simulink model "nn_fuel_control_3_10"  (R2021a)
settings: Solver=ode15s  StartTime=0.0  StopTime=T  MaxStep=.01  RelTol=1e-3
undefined symbols (not defined in the file): AF_sensor_tol, fault_time, fuel_inj_tol, kappa_tol, MAF_sensor_tol, pump_tol, tau_ww_tol
libraries: neural x70
(part 3 of 3)

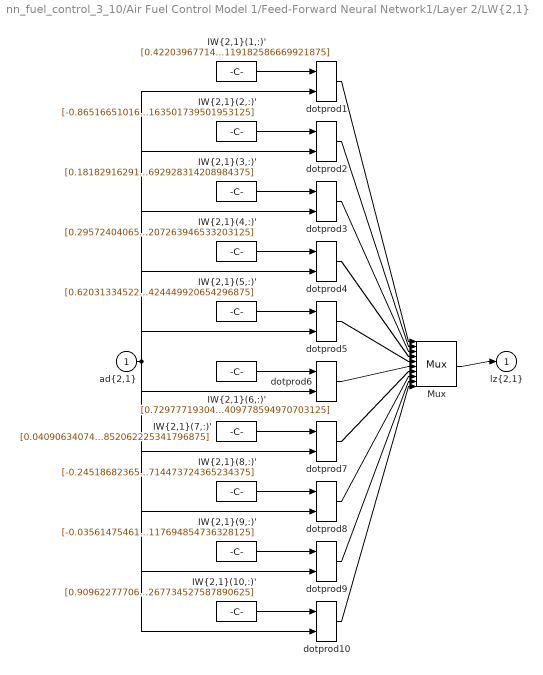
== system nn_fuel_control_3_10/Air Fuel Control Model 1/Feed-Forward Neural Network1/Layer 2/LW{2,1} ==
  "ad{2,1}" : Inport  PortDimensions=10
      mask Display: e = 0.06;c1 = [120 230 180]/255;c2 = ([120 230 180]+0)/(256+128);c3 = ([120 230 180]+128)/(256+128);patch([0 1 1 0],[0 0 1 1],c1);patch([0 1 1 1-e 1-e 0+e],[0 0 1 1-e 0+e 0+e],c2);patch([0 0 1 1-e 0+e 0+e],[0 1 1 1-e 1-e 0+e],c3);plot([0 1 1 0 0],[0 0 1 1 0]);
  "IW{2,1}(1,:)'" : Constant  Value=[0.422039677146083092029726913096965290606021881103515625;-0.110092252616240227069965840200893580913543701171875;-0.26250402610766976341238887471263296902179718017578125;-0.0048946197898318555274954633205197751522064208984375;-0.32867619613755272300892329440102912485599517822265625;0.902942789239071341711451168521307408809661865234375;0.4878626703089585792127991226152516901493072509765625;0.617102583012261174388868312234990298748016357421875;0.733631816964918304080356392660178244113922119140625;0.394170838499643849672793294303119182586669921875]
      mask Display: e = 0.06;c1 = [120 150 230]/255;c2 = ([120 150 230]+0)/383;c3 = ([120 150 230]+128)/383;patch([0 1 1 0],[0 0 1 1],c1);patch([0 1 1 1-e 1-e 0+e],[0 0 1 1-e 0+e 0+e],c2);patch([0 0 1 1-e 0+e 0+e],[0 1 1 1-e 1-e 0+e],c3);plot([0 1 1 0 0],[0 0 1 1 0]);disp('weights');
  "IW{2,1}(10,:)'" : Constant  Value=[0.90962277706535576982105339993722736835479736328125;-0.6963449514150970021120201636222191154956817626953125;0.01080664673637077299872544244863092899322509765625;0.3356832194814760583767565549351274967193603515625;-0.8333879786409565948446243055514059960842132568359375;0.0388654008517956839341422892175614833831787109375;-0.876991458324715811301075518713332712650299072265625;0.2552200485621887171561184004531241953372955322265625;0.439737074727967414133900092565454542636871337890625;-0.454907616285860516569528044783510267734527587890625]
      mask Display: e = 0.06;c1 = [120 150 230]/255;c2 = ([120 150 230]+0)/383;c3 = ([120 150 230]+128)/383;patch([0 1 1 0],[0 0 1 1],c1);patch([0 1 1 1-e 1-e 0+e],[0 0 1 1-e 0+e 0+e],c2);patch([0 0 1 1-e 0+e 0+e],[0 1 1 1-e 1-e 0+e],c3);plot([0 1 1 0 0],[0 0 1 1 0]);disp('weights');
  "IW{2,1}(2,:)'" : Constant  Value=[-0.8651665101614505193339255129103548824787139892578125;-0.68113174408582732866079822997562587261199951171875;0.8404892436305388958572848423500545322895050048828125;0.6586664029004605236394809253397397696971893310546875;-0.7731369627331130534031444767606444656848907470703125;-0.8362478809265689871921267695142887532711029052734375;0.81195057507577839128742880347999744117259979248046875;0.64588522595887110089307725502294488251209259033203125;-0.1523813423040767389693428413011133670806884765625;0.9829939123414395130140519540873356163501739501953125]
      mask Display: e = 0.06;c1 = [120 150 230]/255;c2 = ([120 150 230]+0)/383;c3 = ([120 150 230]+128)/383;patch([0 1 1 0],[0 0 1 1],c1);patch([0 1 1 1-e 1-e 0+e],[0 0 1 1-e 0+e 0+e],c2);patch([0 0 1 1-e 0+e 0+e],[0 1 1 1-e 1-e 0+e],c3);plot([0 1 1 0 0],[0 0 1 1 0]);disp('weights');
  "IW{2,1}(3,:)'" : Constant  Value=[0.181829162913355713016017034533433616161346435546875;-0.881434984567488921669564660987816751003265380859375;-0.1876417286710629905854830212774686515331268310546875;-0.8571525749339719002506399192498065531253814697265625;-0.482981460609078538936955737881362438201904296875;0.56940545520623420117090063286013901233673095703125;0.0259222786987063358310479088686406612396240234375;0.4738233938363729524922973723732866346836090087890625;-0.040986332132006086936826250166632235050201416015625;-0.8081043995213919028941518263309262692928314208984375]
      mask Display: e = 0.06;c1 = [120 150 230]/255;c2 = ([120 150 230]+0)/383;c3 = ([120 150 230]+128)/383;patch([0 1 1 0],[0 0 1 1],c1);patch([0 1 1 1-e 1-e 0+e],[0 0 1 1-e 0+e 0+e],c2);patch([0 0 1 1-e 0+e 0+e],[0 1 1 1-e 1-e 0+e],c3);plot([0 1 1 0 0],[0 0 1 1 0]);disp('weights');
  "IW{2,1}(4,:)'" : Constant  Value=[0.295724040659893938620683684348477981984615325927734375;-0.3268515229616741901708110162871889770030975341796875;-0.279057639543601521125992803717963397502899169921875;0.79686882507062062330760454642586410045623779296875;0.0661197066964048507653473052414483390748500823974609375;-0.63298798947408829729255330676096491515636444091796875;0.1316826637177681558199537903419695794582366943359375;-0.1431159471639171509860233300059917382895946502685546875;0.9243644520376523843196991947479546070098876953125;-0.71110368735452045285683198017068207263946533203125]
      mask Display: e = 0.06;c1 = [120 150 230]/255;c2 = ([120 150 230]+0)/383;c3 = ([120 150 230]+128)/383;patch([0 1 1 0],[0 0 1 1],c1);patch([0 1 1 1-e 1-e 0+e],[0 0 1 1-e 0+e 0+e],c2);patch([0 0 1 1-e 0+e 0+e],[0 1 1 1-e 1-e 0+e],c3);plot([0 1 1 0 0],[0 0 1 1 0]);disp('weights');
  "IW{2,1}(5,:)'" : Constant  Value=[0.6203133452260793934129878834937699139118194580078125;0.901635231669291048461900572874583303928375244140625;-0.3287366297786744606668207779875956475734710693359375;-0.1271174786615658636179659879417158663272857666015625;-0.8464951772599962342980006724246777594089508056640625;0.28518177033808012055260405759327113628387451171875;0.513679542182248649595521783339790999889373779296875;0.6428584550354512483494318075827322900295257568359375;-0.4251606596384103209373961362871341407299041748046875;-0.27453898190018133362855223822407424449920654296875]
      mask Display: e = 0.06;c1 = [120 150 230]/255;c2 = ([120 150 230]+0)/383;c3 = ([120 150 230]+128)/383;patch([0 1 1 0],[0 0 1 1],c1);patch([0 1 1 1-e 1-e 0+e],[0 0 1 1-e 0+e 0+e],c2);patch([0 0 1 1-e 0+e 0+e],[0 1 1 1-e 1-e 0+e],c3);plot([0 1 1 0 0],[0 0 1 1 0]);disp('weights');
  "IW{2,1}(6,:)'" : Constant  Value=[0.7297771930479635127397841642959974706172943115234375;0.23165854469143543070686064311303198337554931640625;0.96494142671238758435237059529754333198070526123046875;-0.390555914482942245768981592846103012561798095703125;-0.90514919206743993385089197545312345027923583984375;-0.438431277886345449612548463846906088292598724365234375;-0.0802142409019130919745066421455703675746917724609375;0.575344599813421897493981305160559713840484619140625;0.1934076537033260212439245151472277939319610595703125;0.934934713944724382628237435710616409778594970703125]
      mask Display: e = 0.06;c1 = [120 150 230]/255;c2 = ([120 150 230]+0)/383;c3 = ([120 150 230]+128)/383;patch([0 1 1 0],[0 0 1 1],c1);patch([0 1 1 1-e 1-e 0+e],[0 0 1 1-e 0+e 0+e],c2);patch([0 0 1 1-e 0+e 0+e],[0 1 1 1-e 1-e 0+e],c3);plot([0 1 1 0 0],[0 0 1 1 0]);disp('weights');
  "IW{2,1}(7,:)'" : Constant  Value=[0.040906340743202616871965204836669727228581905364990234375;0.3152445102858461023487279817345552146434783935546875;-0.96641677936879866184227694247965700924396514892578125;0.858094101605435977120350798941217362880706787109375;0.50777822108413539492488553150906227529048919677734375;-0.19512639085175231823399144559516571462154388427734375;-0.66692474021244618764825418111286126077175140380859375;0.280350917189209847268926978358649648725986480712890625;-0.696901686135316111858628573827445507049560546875;0.326149132414730313911377379554323852062225341796875]
      mask Display: e = 0.06;c1 = [120 150 230]/255;c2 = ([120 150 230]+0)/383;c3 = ([120 150 230]+128)/383;patch([0 1 1 0],[0 0 1 1],c1);patch([0 1 1 1-e 1-e 0+e],[0 0 1 1-e 0+e 0+e],c2);patch([0 0 1 1-e 0+e 0+e],[0 1 1 1-e 1-e 0+e],c3);plot([0 1 1 0 0],[0 0 1 1 0]);disp('weights');
  "IW{2,1}(8,:)'" : Constant  Value=[-0.245186823656732055809470693930052220821380615234375;0.2891152018195357609187112757354043424129486083984375;0.743202086592667843234494284843094646930694580078125;0.3425737123726282362667916459031403064727783203125;-0.057163964796326904860279682907275855541229248046875;-0.3148850353591388095964020976680330932140350341796875;-0.160467488716616646371448950958438217639923095703125;-0.9476340821065243336107641880516894161701202392578125;0.223274479885884336027856988948769867420196533203125;-0.993767070952779274506383444531820714473724365234375]
      mask Display: e = 0.06;c1 = [120 150 230]/255;c2 = ([120 150 230]+0)/383;c3 = ([120 150 230]+128)/383;patch([0 1 1 0],[0 0 1 1],c1);patch([0 1 1 1-e 1-e 0+e],[0 0 1 1-e 0+e 0+e],c2);patch([0 0 1 1-e 0+e 0+e],[0 1 1 1-e 1-e 0+e],c3);plot([0 1 1 0 0],[0 0 1 1 0]);disp('weights');
  "IW{2,1}(9,:)'" : Constant  Value=[-0.035614754618427287014004178899995167739689350128173828125;0.1634174485713522084751048168982379138469696044921875;-0.03107010615764423111517800180081394501030445098876953125;-0.0735264940139603861979367138701491057872772216796875;0.455642930383942879046799134812317788600921630859375;-0.70351463548461057317950917422422207891941070556640625;0.04472929077745153858547411118706804700195789337158203125;-0.77337147245237236603543351520784199237823486328125;-0.103734070298024949607906819437630474567413330078125;-0.556461539732368226651715303887613117694854736328125]
      mask Display: e = 0.06;c1 = [120 150 230]/255;c2 = ([120 150 230]+0)/383;c3 = ([120 150 230]+128)/383;patch([0 1 1 0],[0 0 1 1],c1);patch([0 1 1 1-e 1-e 0+e],[0 0 1 1-e 0+e 0+e],c2);patch([0 0 1 1-e 0+e 0+e],[0 1 1 1-e 1-e 0+e],c3);plot([0 1 1 0 0],[0 0 1 1 0]);disp('weights');
  Mux : Mux  Inputs=10
      mask Display: e = 0.06;c1 = [120 150 230]/255;c2 = ([120 150 230]+0)/383;c3 = ([120 150 230]+128)/383;patch([0 1 1 0],[0 0 1 1],c1);patch([0 1 1 1-e 1-e 0+e],[0 0 1 1-e 0+e 0+e],c2);patch([0 0 1 1-e 0+e 0+e],[0 1 1 1-e 1-e 0+e],c3);plot([0 1 1 0 0],[0 0 1 1 0]);disp('Mux');
  dotprod{1..10} (10 alike) : neural/Weight Functions/dotprod
  "lz{2,1}" : Outport
      mask Display: e = 0.06;c1 = [120 230 180]/255;c2 = ([120 230 180]+0)/(256+128);c3 = ([120 230 180]+128)/(256+128);patch([0 1 1 0],[0 0 1 1],c1);patch([0 1 1 1-e 1-e 0+e],[0 0 1 1-e 0+e 0+e],c2);patch([0 0 1 1-e 0+e 0+e],[0 1 1 1-e 1-e 0+e],c3);plot([0 1 1 0 0],[0 0 1 1 0]);
  wires:
  "IW{2,1}(1,:)'"/1 -> dotprod1/1
  "ad{2,1}"/1 -> dotprod1/2, dotprod2/2, dotprod3/2, dotprod4/2, dotprod5/2, dotprod6/2, dotprod7/2, dotprod8/2, dotprod9/2, dotprod10/2
  dotprod1/1 -> Mux/1
  "IW{2,1}(2,:)'"/1 -> dotprod2/1
  dotprod2/1 -> Mux/2
  "IW{2,1}(3,:)'"/1 -> dotprod3/1
  dotprod3/1 -> Mux/3
  "IW{2,1}(4,:)'"/1 -> dotprod4/1
  dotprod4/1 -> Mux/4
  "IW{2,1}(5,:)'"/1 -> dotprod5/1
  dotprod5/1 -> Mux/5
  "IW{2,1}(6,:)'"/1 -> dotprod6/1
  dotprod6/1 -> Mux/6
  "IW{2,1}(7,:)'"/1 -> dotprod7/1
  dotprod7/1 -> Mux/7
  "IW{2,1}(8,:)'"/1 -> dotprod8/1
  dotprod8/1 -> Mux/8
  "IW{2,1}(9,:)'"/1 -> dotprod9/1
  dotprod9/1 -> Mux/9
  "IW{2,1}(10,:)'"/1 -> dotprod10/1
  dotprod10/1 -> Mux/10
  Mux/1 -> "lz{2,1}"/1

== system nn_fuel_control_3_10/Air Fuel Control Model 1/Feed-Forward Neural Network1/Layer 3/Delays 1 ==
  "p{3}" : Inport  PortDimensions=10
      mask Display: e = 0.06;c1 = [120 230 180]/255;c2 = ([120 230 180]+0)/(256+128);c3 = ([120 230 180]+128)/(256+128);patch([0 1 1 0],[0 0 1 1],c1);patch([0 1 1 1-e 1-e 0+e],[0 0 1 1-e 0+e 0+e],c2);patch([0 0 1 1-e 0+e 0+e],[0 1 1 1-e 1-e 0+e],c3);plot([0 1 1 0 0],[0 0 1 1 0]);
  mux : Mux  Inputs=1
      mask Display: e = 0.06;c1 = [120 150 230]/255;c2 = ([120 150 230]+0)/383;c3 = ([120 150 230]+128)/383;patch([0 1 1 0],[0 0 1 1],c1);patch([0 1 1 1-e 1-e 0+e],[0 0 1 1-e 0+e 0+e],c2);patch([0 0 1 1-e 0+e 0+e],[0 1 1 1-e 1-e 0+e],c3);plot([0 1 1 0 0],[0 0 1 1 0]);disp('Mux')
  "pd{3,2}" : Outport
      mask Display: e = 0.06;c1 = [120 230 180]/255;c2 = ([120 230 180]+0)/(256+128);c3 = ([120 230 180]+128)/(256+128);patch([0 1 1 0],[0 0 1 1],c1);patch([0 1 1 1-e 1-e 0+e],[0 0 1 1-e 0+e 0+e],c2);patch([0 0 1 1-e 0+e 0+e],[0 1 1 1-e 1-e 0+e],c3);plot([0 1 1 0 0],[0 0 1 1 0]);
  wires:
  "p{3}"/1 -> mux/1
  mux/1 -> "pd{3,2}"/1

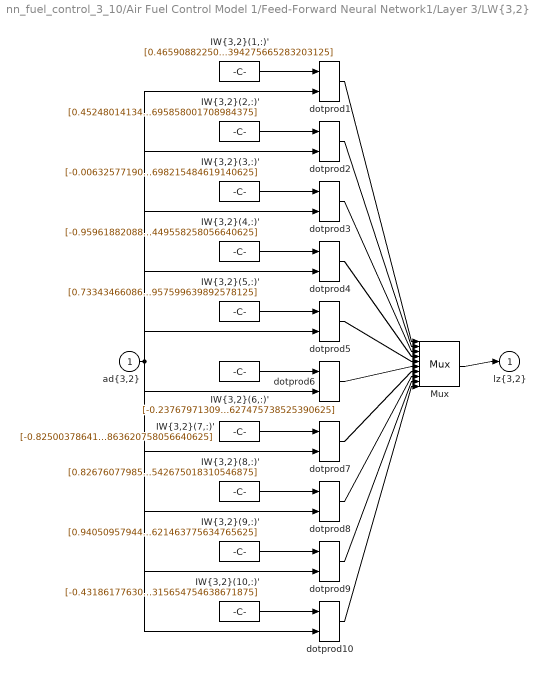
== system nn_fuel_control_3_10/Air Fuel Control Model 1/Feed-Forward Neural Network1/Layer 3/LW{3,2} ==
  "ad{3,2}" : Inport  PortDimensions=10
      mask Display: e = 0.06;c1 = [120 230 180]/255;c2 = ([120 230 180]+0)/(256+128);c3 = ([120 230 180]+128)/(256+128);patch([0 1 1 0],[0 0 1 1],c1);patch([0 1 1 1-e 1-e 0+e],[0 0 1 1-e 0+e 0+e],c2);patch([0 0 1 1-e 0+e 0+e],[0 1 1 1-e 1-e 0+e],c3);plot([0 1 1 0 0],[0 0 1 1 0]);
  "IW{3,2}(1,:)'" : Constant  Value=[0.465908822500017583134734877603477798402309417724609375;-0.413487608206142664979410028536221943795680999755859375;-0.25595023125727589530242767068557441234588623046875;0.79533255427383819924358476782799698412418365478515625;-0.3198554688185104577513584445114247500896453857421875;-0.26425170262540387255967289092950522899627685546875;-0.96446227621692859344193493598140776157379150390625;0.1110265066473614670172764817834831774234771728515625;0.22084634591132246139721928557264618575572967529296875;-0.0783795812571821404191041438025422394275665283203125]
      mask Display: e = 0.06;c1 = [120 150 230]/255;c2 = ([120 150 230]+0)/383;c3 = ([120 150 230]+128)/383;patch([0 1 1 0],[0 0 1 1],c1);patch([0 1 1 1-e 1-e 0+e],[0 0 1 1-e 0+e 0+e],c2);patch([0 0 1 1-e 0+e 0+e],[0 1 1 1-e 1-e 0+e],c3);plot([0 1 1 0 0],[0 0 1 1 0]);disp('weights');
  "IW{3,2}(10,:)'" : Constant  Value=[-0.4318617763054584113291411995305679738521575927734375;-0.032997678117612373738243292109473259188234806060791015625;0.077801025420537239796203721198253333568572998046875;-0.28911309780956695458797867104294709861278533935546875;-0.276713333572291997342063041287474334239959716796875;-0.263564907235820322650710068046464584767818450927734375;-0.51348229867116312874486538930796086788177490234375;-0.6075701084650637628925551325664855539798736572265625;-0.1908663702211096657723743419410311616957187652587890625;0.502134394339247336347398231737315654754638671875]
      mask Display: e = 0.06;c1 = [120 150 230]/255;c2 = ([120 150 230]+0)/383;c3 = ([120 150 230]+128)/383;patch([0 1 1 0],[0 0 1 1],c1);patch([0 1 1 1-e 1-e 0+e],[0 0 1 1-e 0+e 0+e],c2);patch([0 0 1 1-e 0+e 0+e],[0 1 1 1-e 1-e 0+e],c3);plot([0 1 1 0 0],[0 0 1 1 0]);disp('weights');
  "IW{3,2}(2,:)'" : Constant  Value=[0.452480141341178032643455253491993062198162078857421875;0.336080692249946688665573901744210161268711090087890625;-0.750580224709083143608268073876388370990753173828125;-0.52823687812015529541298519689007662236690521240234375;0.602301465570855842912578737013973295688629150390625;0.63024563212891104857504842584603466093540191650390625;-0.356127133216790958680775247557903639972209930419921875;-0.036352884411245955931235585012473165988922119140625;0.291588369681691716994720309230615384876728057861328125;0.1676526656541683646395313189714215695858001708984375]
      mask Display: e = 0.06;c1 = [120 150 230]/255;c2 = ([120 150 230]+0)/383;c3 = ([120 150 230]+128)/383;patch([0 1 1 0],[0 0 1 1],c1);patch([0 1 1 1-e 1-e 0+e],[0 0 1 1-e 0+e 0+e],c2);patch([0 0 1 1-e 0+e 0+e],[0 1 1 1-e 1-e 0+e],c3);plot([0 1 1 0 0],[0 0 1 1 0]);disp('weights');
  "IW{3,2}(3,:)'" : Constant  Value=[-0.0063257719015989977151548373512923717498779296875;0.1558232650998754298399262552266009151935577392578125;0.21356467202521312032104106037877500057220458984375;-0.5606276936605281147052437518141232430934906005859375;0.51247289446128529988300215336494147777557373046875;-0.6789132841767884229966512066312134265899658203125;-0.105704557253306408171056318678893148899078369140625;-0.0089827216141546983863008790649473667144775390625;0.010488749062883329088435857556760311126708984375;0.1097273920785470924244009438552893698215484619140625]
      mask Display: e = 0.06;c1 = [120 150 230]/255;c2 = ([120 150 230]+0)/383;c3 = ([120 150 230]+128)/383;patch([0 1 1 0],[0 0 1 1],c1);patch([0 1 1 1-e 1-e 0+e],[0 0 1 1-e 0+e 0+e],c2);patch([0 0 1 1-e 0+e 0+e],[0 1 1 1-e 1-e 0+e],c3);plot([0 1 1 0 0],[0 0 1 1 0]);disp('weights');
  "IW{3,2}(4,:)'" : Constant  Value=[-0.9596188208888793980122500215657055377960205078125;-0.8746551071446122538333156626322306692600250244140625;-0.1240862576936716532571836069109849631786346435546875;-0.9366084767927647103391564087360166013240814208984375;-0.2263567918631845810040204014512710273265838623046875;-0.7551613682655489157014017109759151935577392578125;-0.0137802781081342029523284509195946156978607177734375;0.978542105587190125248753247433342039585113525390625;-0.1979323813352078520466648114961571991443634033203125;0.636282512328963267833614736446179449558258056640625]
      mask Display: e = 0.06;c1 = [120 150 230]/255;c2 = ([120 150 230]+0)/383;c3 = ([120 150 230]+128)/383;patch([0 1 1 0],[0 0 1 1],c1);patch([0 1 1 1-e 1-e 0+e],[0 0 1 1-e 0+e 0+e],c2);patch([0 0 1 1-e 0+e 0+e],[0 1 1 1-e 1-e 0+e],c3);plot([0 1 1 0 0],[0 0 1 1 0]);disp('weights');
  "IW{3,2}(5,:)'" : Constant  Value=[0.73343466086165565176457903362461365759372711181640625;0.960980758123656908509246932226233184337615966796875;-0.134217532509697701215145571040920913219451904296875;0.11442774545926277796059622460234095342457294464111328125;0.6723741038002055692146541332476772367954254150390625;0.1438551765328461851112251679296605288982391357421875;0.9363889336038428989894555343198589980602264404296875;0.137441760075660557305354814161546528339385986328125;-0.8843285718670441664102099821320734918117523193359375;0.5522017606648639276301082645659334957599639892578125]
      mask Display: e = 0.06;c1 = [120 150 230]/255;c2 = ([120 150 230]+0)/383;c3 = ([120 150 230]+128)/383;patch([0 1 1 0],[0 0 1 1],c1);patch([0 1 1 1-e 1-e 0+e],[0 0 1 1-e 0+e 0+e],c2);patch([0 0 1 1-e 0+e 0+e],[0 1 1 1-e 1-e 0+e],c3);plot([0 1 1 0 0],[0 0 1 1 0]);disp('weights');
  "IW{3,2}(6,:)'" : Constant  Value=[-0.2376797130922718437329166363269905559718608856201171875;-0.3245060471454490613751886485260911285877227783203125;0.411253730585999566216059974976815283298492431640625;0.3281032645082484489051921627833507955074310302734375;-0.5180651518724077586597331901430152356624603271484375;-0.5577078697023740705418504148838110268115997314453125;-0.422261332231368469170007529100985266268253326416015625;-0.070689711751910966341938546975143253803253173828125;-0.1758320370175628089004504772674408741295337677001953125;0.7513529749619716202602148769074119627475738525390625]
      mask Display: e = 0.06;c1 = [120 150 230]/255;c2 = ([120 150 230]+0)/383;c3 = ([120 150 230]+128)/383;patch([0 1 1 0],[0 0 1 1],c1);patch([0 1 1 1-e 1-e 0+e],[0 0 1 1-e 0+e 0+e],c2);patch([0 0 1 1-e 0+e 0+e],[0 1 1 1-e 1-e 0+e],c3);plot([0 1 1 0 0],[0 0 1 1 0]);disp('weights');
  "IW{3,2}(7,:)'" : Constant  Value=[-0.82500378641395910594980023233802057802677154541015625;0.96291679796392204426780381254502572119235992431640625;0.5803596168647000563822757612797431647777557373046875;-0.2701456506325394801848460701876319944858551025390625;0.8890348593138062138763189068413339555263519287109375;0.1501557516428747851566782856025383807718753814697265625;0.481666771587706765700431787990964949131011962890625;-0.7831361801558021085156724439002573490142822265625;-0.026613027462942674683521460110569023527204990386962890625;-0.1646446034291531024251753478893078863620758056640625]
      mask Display: e = 0.06;c1 = [120 150 230]/255;c2 = ([120 150 230]+0)/383;c3 = ([120 150 230]+128)/383;patch([0 1 1 0],[0 0 1 1],c1);patch([0 1 1 1-e 1-e 0+e],[0 0 1 1-e 0+e 0+e],c2);patch([0 0 1 1-e 0+e 0+e],[0 1 1 1-e 1-e 0+e],c3);plot([0 1 1 0 0],[0 0 1 1 0]);disp('weights');
  "IW{3,2}(8,:)'" : Constant  Value=[0.82676077985266804848407673489418812096118927001953125;-0.87879337999093143363182889515883289277553558349609375;-0.8573989414424232347045062851975671947002410888671875;0.6488948308169446566040505786077119410037994384765625;0.841872789003470956004093750379979610443115234375;-0.55549591509967577440676222977344878017902374267578125;0.59327158091704268461086257957504130899906158447265625;0.369291055697225534260041968082077801227569580078125;0.89098865986625153112754560424946248531341552734375;0.945757196895765428479307956877164542675018310546875]
      mask Display: e = 0.06;c1 = [120 150 230]/255;c2 = ([120 150 230]+0)/383;c3 = ([120 150 230]+128)/383;patch([0 1 1 0],[0 0 1 1],c1);patch([0 1 1 1-e 1-e 0+e],[0 0 1 1-e 0+e 0+e],c2);patch([0 0 1 1-e 0+e 0+e],[0 1 1 1-e 1-e 0+e],c3);plot([0 1 1 0 0],[0 0 1 1 0]);disp('weights');
  "IW{3,2}(9,:)'" : Constant  Value=[0.9405095794473343762120975952711887657642364501953125;-0.188806428409112159183536050477414391934871673583984375;0.8350720698739089176143579607014544308185577392578125;0.2144367638571101630784454528111382387578487396240234375;-0.3297992370033802078665985391126014292240142822265625;0.00879039483057554062173100106747369864024221897125244140625;0.66039899729722628674011275506927631795406341552734375;-0.3996949053173801669203157871379517018795013427734375;-0.90049767130397506686989572699530981481075286865234375;-0.0075342401012241655422485564486123621463775634765625]
      mask Display: e = 0.06;c1 = [120 150 230]/255;c2 = ([120 150 230]+0)/383;c3 = ([120 150 230]+128)/383;patch([0 1 1 0],[0 0 1 1],c1);patch([0 1 1 1-e 1-e 0+e],[0 0 1 1-e 0+e 0+e],c2);patch([0 0 1 1-e 0+e 0+e],[0 1 1 1-e 1-e 0+e],c3);plot([0 1 1 0 0],[0 0 1 1 0]);disp('weights');
  Mux : Mux  Inputs=10
      mask Display: e = 0.06;c1 = [120 150 230]/255;c2 = ([120 150 230]+0)/383;c3 = ([120 150 230]+128)/383;patch([0 1 1 0],[0 0 1 1],c1);patch([0 1 1 1-e 1-e 0+e],[0 0 1 1-e 0+e 0+e],c2);patch([0 0 1 1-e 0+e 0+e],[0 1 1 1-e 1-e 0+e],c3);plot([0 1 1 0 0],[0 0 1 1 0]);disp('Mux');
  dotprod{1..10} (10 alike) : neural/Weight Functions/dotprod
  "lz{3,2}" : Outport
      mask Display: e = 0.06;c1 = [120 230 180]/255;c2 = ([120 230 180]+0)/(256+128);c3 = ([120 230 180]+128)/(256+128);patch([0 1 1 0],[0 0 1 1],c1);patch([0 1 1 1-e 1-e 0+e],[0 0 1 1-e 0+e 0+e],c2);patch([0 0 1 1-e 0+e 0+e],[0 1 1 1-e 1-e 0+e],c3);plot([0 1 1 0 0],[0 0 1 1 0]);
  wires:
  "IW{3,2}(1,:)'"/1 -> dotprod1/1
  "ad{3,2}"/1 -> dotprod1/2, dotprod2/2, dotprod3/2, dotprod4/2, dotprod5/2, dotprod6/2, dotprod7/2, dotprod8/2, dotprod9/2, dotprod10/2
  dotprod1/1 -> Mux/1
  "IW{3,2}(2,:)'"/1 -> dotprod2/1
  dotprod2/1 -> Mux/2
  "IW{3,2}(3,:)'"/1 -> dotprod3/1
  dotprod3/1 -> Mux/3
  "IW{3,2}(4,:)'"/1 -> dotprod4/1
  dotprod4/1 -> Mux/4
  "IW{3,2}(5,:)'"/1 -> dotprod5/1
  dotprod5/1 -> Mux/5
  "IW{3,2}(6,:)'"/1 -> dotprod6/1
  dotprod6/1 -> Mux/6
  "IW{3,2}(7,:)'"/1 -> dotprod7/1
  dotprod7/1 -> Mux/7
  "IW{3,2}(8,:)'"/1 -> dotprod8/1
  dotprod8/1 -> Mux/8
  "IW{3,2}(9,:)'"/1 -> dotprod9/1
  dotprod9/1 -> Mux/9
  "IW{3,2}(10,:)'"/1 -> dotprod10/1
  dotprod10/1 -> Mux/10
  Mux/1 -> "lz{3,2}"/1

== system nn_fuel_control_3_10/Air Fuel Control Model 1/Feed-Forward Neural Network1/Layer 4/Delays 1 ==
  "p{4}" : Inport  PortDimensions=10
      mask Display: e = 0.06;c1 = [120 230 180]/255;c2 = ([120 230 180]+0)/(256+128);c3 = ([120 230 180]+128)/(256+128);patch([0 1 1 0],[0 0 1 1],c1);patch([0 1 1 1-e 1-e 0+e],[0 0 1 1-e 0+e 0+e],c2);patch([0 0 1 1-e 0+e 0+e],[0 1 1 1-e 1-e 0+e],c3);plot([0 1 1 0 0],[0 0 1 1 0]);
  mux : Mux  Inputs=1
      mask Display: e = 0.06;c1 = [120 150 230]/255;c2 = ([120 150 230]+0)/383;c3 = ([120 150 230]+128)/383;patch([0 1 1 0],[0 0 1 1],c1);patch([0 1 1 1-e 1-e 0+e],[0 0 1 1-e 0+e 0+e],c2);patch([0 0 1 1-e 0+e 0+e],[0 1 1 1-e 1-e 0+e],c3);plot([0 1 1 0 0],[0 0 1 1 0]);disp('Mux')
  "pd{4,3}" : Outport
      mask Display: e = 0.06;c1 = [120 230 180]/255;c2 = ([120 230 180]+0)/(256+128);c3 = ([120 230 180]+128)/(256+128);patch([0 1 1 0],[0 0 1 1],c1);patch([0 1 1 1-e 1-e 0+e],[0 0 1 1-e 0+e 0+e],c2);patch([0 0 1 1-e 0+e 0+e],[0 1 1 1-e 1-e 0+e],c3);plot([0 1 1 0 0],[0 0 1 1 0]);
  wires:
  "p{4}"/1 -> mux/1
  mux/1 -> "pd{4,3}"/1

== system nn_fuel_control_3_10/Air Fuel Control Model 1/Feed-Forward Neural Network1/Layer 4/LW{4,3} ==
  "ad{4,3}" : Inport  PortDimensions=10
      mask Display: e = 0.06;c1 = [120 230 180]/255;c2 = ([120 230 180]+0)/(256+128);c3 = ([120 230 180]+128)/(256+128);patch([0 1 1 0],[0 0 1 1],c1);patch([0 1 1 1-e 1-e 0+e],[0 0 1 1-e 0+e 0+e],c2);patch([0 0 1 1-e 0+e 0+e],[0 1 1 1-e 1-e 0+e],c3);plot([0 1 1 0 0],[0 0 1 1 0]);
  "IW{4,3}(1,:)'" : Constant  Value=[-1.167925860607833765669738568249158561229705810546875;0.81386441477208848471747160147060640156269073486328125;0.5288555595633328554328045356669463217258453369140625;-0.941477290637221297942005548975430428981781005859375;0.1806444600688257573484207796354894526302814483642578125;0.84162355301070679303165888995863497257232666015625;-0.033721100046846981534987008899406646378338336944580078125;0.2302489645241232174566192725251312367618083953857421875;-0.53788375116973752287918841830105520784854888916015625;0.7619909098526924662309056657250039279460906982421875]
      mask Display: e = 0.06;c1 = [120 150 230]/255;c2 = ([120 150 230]+0)/383;c3 = ([120 150 230]+128)/383;patch([0 1 1 0],[0 0 1 1],c1);patch([0 1 1 1-e 1-e 0+e],[0 0 1 1-e 0+e 0+e],c2);patch([0 0 1 1-e 0+e 0+e],[0 1 1 1-e 1-e 0+e],c3);plot([0 1 1 0 0],[0 0 1 1 0]);disp('weights');
  Mux : Mux  Inputs=1
      mask Display: e = 0.06;c1 = [120 150 230]/255;c2 = ([120 150 230]+0)/383;c3 = ([120 150 230]+128)/383;patch([0 1 1 0],[0 0 1 1],c1);patch([0 1 1 1-e 1-e 0+e],[0 0 1 1-e 0+e 0+e],c2);patch([0 0 1 1-e 0+e 0+e],[0 1 1 1-e 1-e 0+e],c3);plot([0 1 1 0 0],[0 0 1 1 0]);disp('Mux');
  dotprod1 : neural/Weight Functions/dotprod
  "lz{4,3}" : Outport
      mask Display: e = 0.06;c1 = [120 230 180]/255;c2 = ([120 230 180]+0)/(256+128);c3 = ([120 230 180]+128)/(256+128);patch([0 1 1 0],[0 0 1 1],c1);patch([0 1 1 1-e 1-e 0+e],[0 0 1 1-e 0+e 0+e],c2);patch([0 0 1 1-e 0+e 0+e],[0 1 1 1-e 1-e 0+e],c3);plot([0 1 1 0 0],[0 0 1 1 0]);
  wires:
  "IW{4,3}(1,:)'"/1 -> dotprod1/1
  "ad{4,3}"/1 -> dotprod1/2
  dotprod1/1 -> Mux/1
  Mux/1 -> "lz{4,3}"/1
